simulink model "MachineOne"  (R2022a)
settings: Solver=FixedStepAuto  StartTime=0.0  StopTime=inf  RelTol=1e-3  EnableMultiTasking=on
libraries: arduinolib x1
settings Model: ExtModeTrigDuration=2  Creator=nikhi  LastModifiedBy=Lagadh Matsa
settings SolverCC: AlgebraicLoopSolver=TrustRegion
settings OptimizationCC: EnhancedBackFolding=on  PassReuseOutputArgsThreshold=0  MaxStackSize=64  OptimizeBlockOrder=speed  DifferentSizesBufferReuse=on  OptimizationCustomize=off
settings DebuggingCC: ParameterTunabilityLossMsg=error  UnconnectedInputMsg=warning  UnconnectedOutputMsg=warning  UnconnectedLineMsg=warning  SFMachineParentedDataDiag=warning
settings HardwareCC: ProdBitPerInt=16  ProdBitPerPointer=16  ProdBitPerSizeT=16  ProdBitPerPtrDiffT=16  ProdLargestAtomicFloat=None  ProdWordSize=8  ProdHWDeviceType=Atmel->AVR  UseEmbeddedCoderFeatures=off  UseSimulinkCoderFeatures=off
settings SFSimCC: MATLABDynamicMemAlloc=off
settings RTWCC: SystemTargetFile=ert.tlc  HardwareBoard=Arduino Uno  TemplateMakefile=ert_default_tmf  Toolchain=Arduino AVR  BuildConfiguration=Faster Runs  DLArmComputeVersion=19.05
settings CodeAppCC: ForceParamTrailComments=on  OperatorAnnotations=on
settings ERTTargetCC: ERTCustomFileBanners=off  SupportContinuousTime=on  SupportNonInlinedSFcns=on  RemoveResetFunc=off  SupportVariableSizeSignals=on  ModelStepFunctionPrototypeControlCompliant=off  ExtModeStaticAllocSize=250

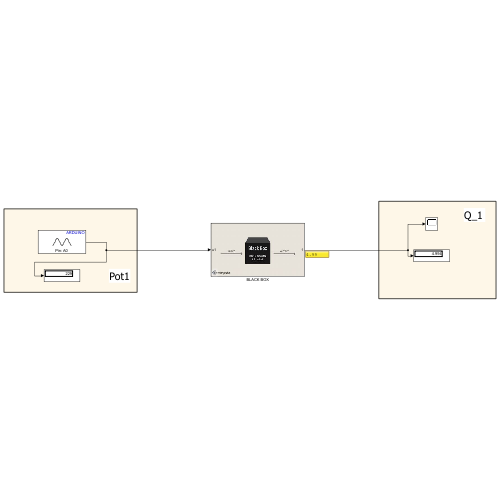
[thumbnail: Simulink's stored preview of the top-level diagram]
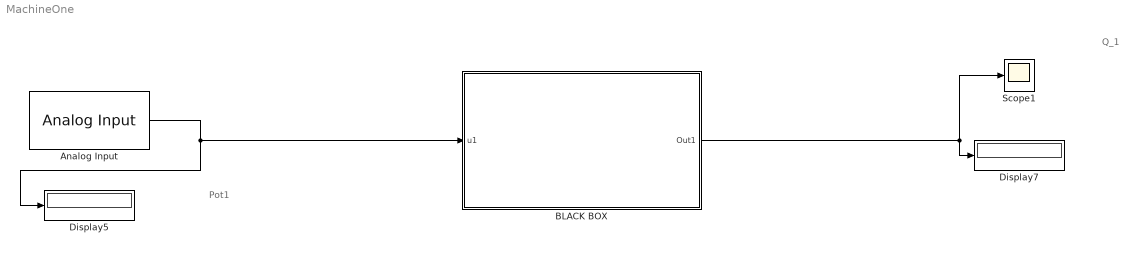
== system MachineOne ==
  note: Q_1
  note: Pot1
  Analog Input : arduinolib/Analog Input  pinNumber=0  ReadResultsOnly=off  ConversionTriggerSource=Software  ExternalTriggerType=uint32( 0 )  OutputDataType=uint16  EnableConversionCompleteNotify=off  EnableOuputStatus=off  SampleTime=1  blockPlatform=arduino
  BLACK BOX : Subsystem
      mask Display: image('1.jfif'); % Use "Edit Image" on toolstrip to change.
  Display5 : Display
  Display7 : Display
  Scope1 : Scope
  wires:
  Analog Input/1 -> Display5/1, BLACK BOX/1(u1)
  BLACK BOX/1(Out1) -> Scope1/1, Display7/1

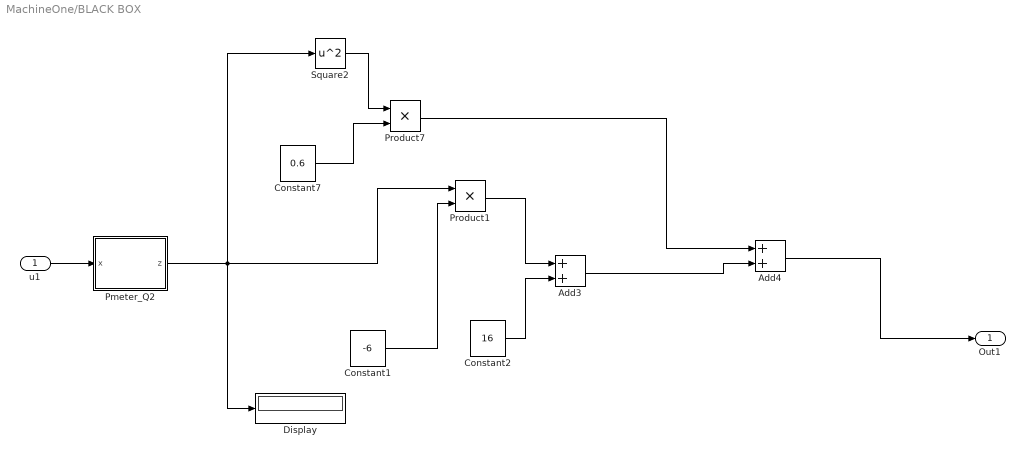
== system MachineOne/BLACK BOX ==
  u1 : Inport
  Add3 : Sum
  Add4 : Sum
  Constant1 : Constant  Value=-6
  Constant2 : Constant  Value=16
  Constant7 : Constant  Value=0.6
  Display : Display
  Pmeter_Q2 : MATLAB Function  TreatAsAtomicUnit=on
  Product1 : Product
  Product7 : Product
  Square2 : Math  Operator=square
  Out1 : Outport
  wires:
  Add3/1 -> Add4/2
  Add4/1 -> Out1/1
  Constant7/1 -> Product7/2
  Pmeter_Q2/1(z) -> Display/1, Product1/1, Square2/1
  u1/1 -> Pmeter_Q2/1(x)
  Square2/1 -> Product7/1
  Constant1/1 -> Product1/2
  Product1/1 -> Add3/1
  Constant2/1 -> Add3/2
  Product7/1 -> Add4/1

== matlab function MachineOne/BLACK BOX/Pmeter_Q2 ==
  data: x input; z output
function z = fcn(x)
z = 0;
if x > 250 & x < 770
    z = (double(x)*0.01);
else
    z = double(7.58);
end
z = z;
